simulink model "BIT8_COMP"  (R2019b)
settings: Solver=ode8  StartTime=0.0  StopTime=9999  FixedStep=1  RelTol=1e-3
values from neighbouring files (symbols this model uses):
  CODE = [ ... (first row only)    [ATE_BIT_SCRIPTS.m]
libraries: TURING_LOGIC x44, NOT x2
settings Model: EnablePacing=on  Creator=JTHURT  LastModifiedBy=JTHURT
settings DebuggingCC: SFMachineParentedDataDiag=error

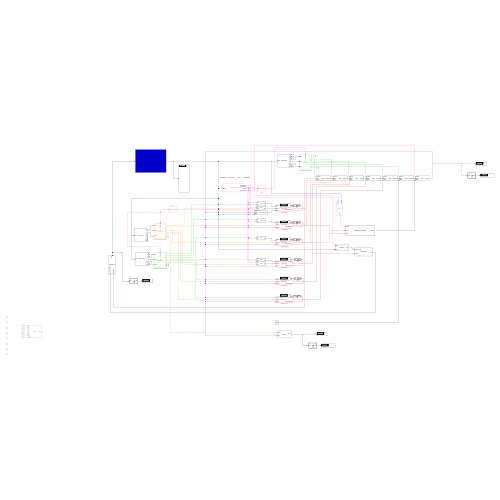
[thumbnail: Simulink's stored preview of the top-level diagram]
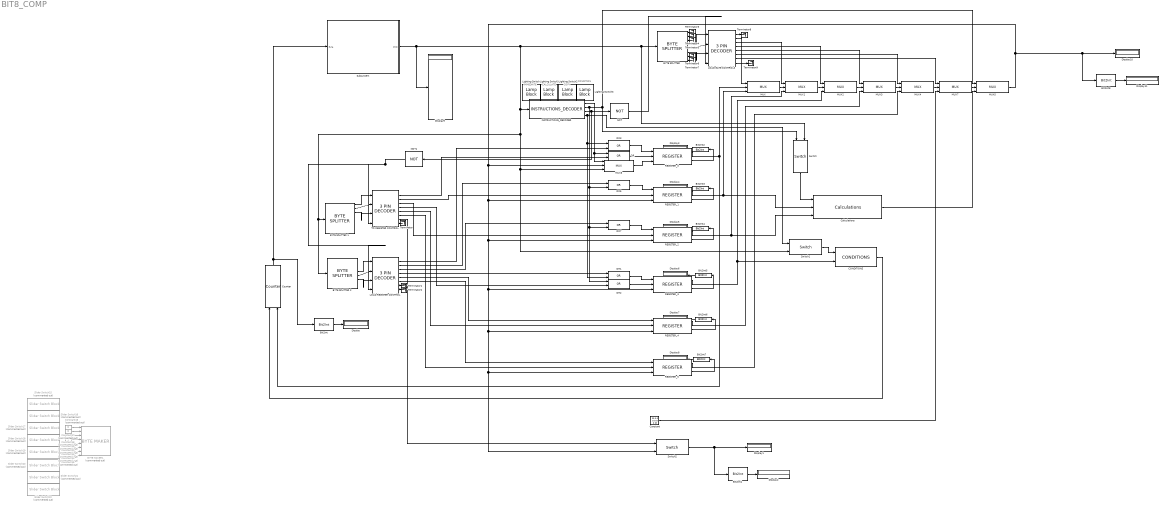
== system BIT8_COMP ==
  note: CONDITION
  note: COPY
  note: CALCULATE
  note: IMMEDIATE
  BYTE MAKER1 : TURING_LOGIC/BYTE MAKER  Commented=on  SystemSampleTime=-1  Latency=0  AutoFrameSizeCalculation=off
      settings: SourceProductName=Turing Logic
  "BYTE SPLITTER " : TURING_LOGIC/BYTE SPLITTER   SystemSampleTime=-1  Latency=0  AutoFrameSizeCalculation=off
      settings: SourceProductName=Turing Logic
  BYTE SPLITTER 1 : TURING_LOGIC/BYTE SPLITTER   SystemSampleTime=-1  Latency=0  AutoFrameSizeCalculation=off
      settings: SourceProductName=Turing Logic
  BYTE SPLITTER 2 : TURING_LOGIC/BYTE SPLITTER   SystemSampleTime=-1  Latency=0  AutoFrameSizeCalculation=off
      settings: SourceProductName=Turing Logic
  Bit2Int{,1..8} (9 alike) : TURING_LOGIC/Bit2Int  SystemSampleTime=-1  Latency=0  AutoFrameSizeCalculation=off
      settings: SourceProductName=Turing Logic
  CONDITIONS : TURING_LOGIC/CONDITIONS  SystemSampleTime=-1  Latency=0  AutoFrameSizeCalculation=off
      settings: SourceProductName=Turing Logic
  Calculations : TURING_LOGIC/Calculations  SystemSampleTime=-1  Latency=0  AutoFrameSizeCalculation=off
      settings: SourceProductName=Turing Logic
  Constant : Constant  Value=[0 0 0 0 0 0 0 0]  SampleTime=-1
  Constant{13..14,16..18,20} (6 alike) : Constant  Commented=on  Value=0  SampleTime=-1
  Constant15 : Constant  Commented=on  SampleTime=-1
  Constant19 : Constant  Commented=on  SampleTime=-1
  Counter : TURING_LOGIC/Counter  SystemSampleTime=-1  Latency=0  AutoFrameSizeCalculation=off
      settings: SourceProductName=Turing Logic
  Display{,1..11} (12 alike) : Display
  INSTRUCTIONS_DECODER : TURING_LOGIC/INSTRUCTIONS_DECODER  SystemSampleTime=-1  Latency=0  AutoFrameSizeCalculation=off
      settings: SourceProductName=Turing Logic
  LOAD GATE CONTROLS : TURING_LOGIC/3 PIN DECODER  SystemSampleTime=-1  Latency=0  AutoFrameSizeCalculation=off
      settings: SourceProductName=Turing Logic
  LOAD REGISTER CONTROL : TURING_LOGIC/3 PIN DECODER  SystemSampleTime=-1  Latency=0  AutoFrameSizeCalculation=off
      settings: SourceProductName=Turing Logic
  Lighting Switch{,1..3} (4 alike) : LampBlock  LabelPosition=Hide  Icon=LightingSwitch
  MUX{,1..7} (8 alike) : TURING_LOGIC/MUX  SystemSampleTime=-1  Latency=0  AutoFrameSizeCalculation=off
      settings: SourceProductName=Turing Logic
  NOT : NOT/NOT  SystemSampleTime=-1  Latency=0  AutoFrameSizeCalculation=off
  NOT1 : NOT/NOT  SystemSampleTime=-1  Latency=0  AutoFrameSizeCalculation=off
  OR{,1..3,5,7} (6 alike) : TURING_LOGIC/OR  SystemSampleTime=-1  Latency=0  AutoFrameSizeCalculation=off
      settings: SourceProductName=Turing Logic
  REGISTER_{0..5} (6 alike) : TURING_LOGIC/REGISTER  SystemSampleTime=-1  Latency=0  AutoFrameSizeCalculation=off
      settings: SourceProductName=Turing Logic
  Slider Switch{15..22} (8 alike) : SliderSwitchBlock  Commented=on
      settings: Values={{'Off', 'On'}, [0 1]}
  Subsystem : Subsystem
  Switch : TURING_LOGIC/Switch  SystemSampleTime=-1  Latency=0  AutoFrameSizeCalculation=off
      settings: SourceProductName=Turing Logic
  Switch1 : TURING_LOGIC/Switch  SystemSampleTime=-1  Latency=0  AutoFrameSizeCalculation=off
      settings: SourceProductName=Turing Logic
  Switch2 : TURING_LOGIC/Switch  SystemSampleTime=-1  Latency=0  AutoFrameSizeCalculation=off
      settings: SourceProductName=Turing Logic
  TO REGISTER CONTROL : TURING_LOGIC/3 PIN DECODER  SystemSampleTime=-1  Latency=0  AutoFrameSizeCalculation=off
      settings: SourceProductName=Turing Logic
  Terminator{,1..9} (10 alike) : Terminator
  wires:
  Counter/1 -> Bit2Int/1, Subsystem/1(Byte)
  Subsystem/1(CMD) -> Display9/1, Switch/2, "BYTE SPLITTER "/1, BYTE SPLITTER 2/1, BYTE SPLITTER 1/1, MUX6/3, Switch1/2, INSTRUCTIONS_DECODER/1
  "BYTE SPLITTER "/4 -> LOAD GATE CONTROLS/1
  "BYTE SPLITTER "/5 -> LOAD GATE CONTROLS/2
  "BYTE SPLITTER "/6 -> LOAD GATE CONTROLS/3
  MUX/1 -> MUX1/2
  MUX1/1 -> MUX2/2
  MUX2/1 -> MUX3/2
  MUX3/1 -> MUX4/2
  LOAD GATE CONTROLS/2 -> MUX/1
  LOAD GATE CONTROLS/3 -> MUX1/1
  LOAD GATE CONTROLS/4 -> MUX2/1
  LOAD GATE CONTROLS/5 -> MUX3/1
  LOAD GATE CONTROLS/6 -> MUX4/1
  BYTE SPLITTER 1/1 -> TO REGISTER CONTROL/1
  BYTE SPLITTER 1/2 -> TO REGISTER CONTROL/2
  BYTE SPLITTER 1/3 -> TO REGISTER CONTROL/3
  BYTE SPLITTER 2/4 -> LOAD REGISTER CONTROL/1
  BYTE SPLITTER 2/5 -> LOAD REGISTER CONTROL/2
  BYTE SPLITTER 2/6 -> LOAD REGISTER CONTROL/3
  OR/1 -> REGISTER_0/2
  INSTRUCTIONS_DECODER/1 -> MUX6/1, OR/1
  TO REGISTER CONTROL/1 -> OR/2
  MUX6/1 -> REGISTER_0/3
  OR5/1 -> REGISTER_1/1
  TO REGISTER CONTROL/2 -> REGISTER_1/2
  TO REGISTER CONTROL/3 -> REGISTER_2/2
  OR7/1 -> REGISTER_2/1
  OR2/1 -> REGISTER_3/2
  OR1/1 -> REGISTER_3/1
  INSTRUCTIONS_DECODER/2 -> OR2/1, OR7/2, OR5/2, MUX5/1, Switch/1
  TO REGISTER CONTROL/4 -> OR2/2
  TO REGISTER CONTROL/5 -> REGISTER_4/2
  TO REGISTER CONTROL/6 -> REGISTER_5/2
  LOAD REGISTER CONTROL/2 -> OR5/1
  LOAD REGISTER CONTROL/3 -> OR7/1
  LOAD REGISTER CONTROL/4 -> OR1/1
  LOAD REGISTER CONTROL/5 -> REGISTER_4/1
  LOAD REGISTER CONTROL/6 -> REGISTER_5/1
  REGISTER_0/1 -> Counter/2, MUX/2
  REGISTER_4/1 -> MUX3/3
  REGISTER_5/1 -> MUX4/3
  INSTRUCTIONS_DECODER/3 -> NOT1/1, NOT/1
  NOT/1 -> LOAD GATE CONTROLS/4
  Switch/1 -> Calculations/1
  Constant20/1 -> BYTE MAKER1/5
  Constant15/1 -> BYTE MAKER1/8
  Constant17/1 -> BYTE MAKER1/2
  Constant19/1 -> BYTE MAKER1/4
  Constant13/1 -> BYTE MAKER1/6
  Constant18/1 -> BYTE MAKER1/3
  Constant16/1 -> BYTE MAKER1/1
  Constant14/1 -> BYTE MAKER1/7
  MUX4/1 -> MUX7/2
  LOAD GATE CONTROLS/7 -> MUX7/1
  MUX7/1 -> MUX5/2
  Calculations/1 -> MUX5/3
  Switch1/1 -> CONDITIONS/1
  INSTRUCTIONS_DECODER/4 -> OR1/2, OR3/1, Switch1/1
  CONDITIONS/1 -> Counter/1
  OR3/1 -> REGISTER_0/1
  LOAD REGISTER CONTROL/1 -> OR3/2
  Constant/1 -> MUX7/3
  TO REGISTER CONTROL/7 -> Switch2/1
  Bit2Int/1 -> Display/1
  Switch2/1 -> Bit2Int1/1, Display1/1
  Bit2Int1/1 -> Display2/1
  Bit2Int2/1 -> Display3/1
  REGISTER_1/1 -> Calculations/2, MUX/3
  Bit2Int3/1 -> Display4/1
  REGISTER_2/1 -> Calculations/3, MUX1/3
  Bit2Int4/1 -> Display5/1
  Bit2Int5/1 -> Display6/1
  REGISTER_3/1 -> CONDITIONS/2, MUX2/3
  Bit2Int6/1 -> Display7/1
  Bit2Int7/1 -> Display8/1
  Bit2Int8/1 -> Display11/1
  MUX5/1 -> Bit2Int8/1, Display10/1, MUX6/2, REGISTER_2/3, REGISTER_4/3, Switch2/2, REGISTER_5/3, REGISTER_3/3, REGISTER_1/3
  REGISTER_0/2 -> Bit2Int2/1
  REGISTER_1/2 -> Bit2Int3/1
  REGISTER_2/2 -> Bit2Int4/1
  REGISTER_3/2 -> Bit2Int5/1
  REGISTER_4/2 -> Bit2Int6/1
  REGISTER_5/2 -> Bit2Int7/1
  NOT1/1 -> LOAD REGISTER CONTROL/4, TO REGISTER CONTROL/4
  TO REGISTER CONTROL/8 -> Terminator/1
  LOAD REGISTER CONTROL/7 -> Terminator1/1
  LOAD REGISTER CONTROL/8 -> Terminator2/1
  "BYTE SPLITTER "/1 -> Terminator3/1
  "BYTE SPLITTER "/2 -> Terminator4/1
  "BYTE SPLITTER "/3 -> Terminator5/1
  "BYTE SPLITTER "/7 -> Terminator6/1
  "BYTE SPLITTER "/8 -> Terminator7/1
  LOAD GATE CONTROLS/1 -> Terminator8/1
  LOAD GATE CONTROLS/8 -> Terminator9/1

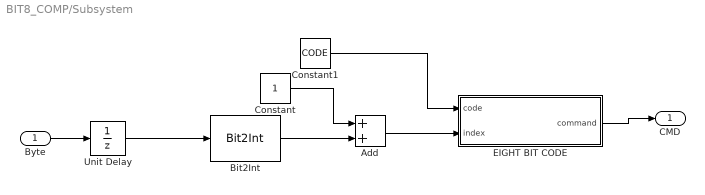
== system BIT8_COMP/Subsystem ==
  Byte : Inport
  Add : Sum
  Bit2Int : TURING_LOGIC/Bit2Int  SystemSampleTime=-1  Latency=0  AutoFrameSizeCalculation=off
      settings: SourceProductName=Turing Logic
  Constant : Constant  SampleTime=-1
  Constant1 : Constant  Value=CODE  SampleTime=-1
  EIGHT BIT CODE : MATLAB Function  TreatAsAtomicUnit=on
  Unit Delay : UnitDelay  InitialCondition=[0 0 0 0 0 0 0 0]  SampleTime=-1  HasFrameUpgradeWarning=on
  CMD : Outport
  wires:
  EIGHT BIT CODE/1(command) -> CMD/1
  Constant/1 -> Add/1
  Add/1 -> EIGHT BIT CODE/2(index)
  Constant1/1 -> EIGHT BIT CODE/1(code)
  Bit2Int/1 -> Add/2
  Byte/1 -> Unit Delay/1
  Unit Delay/1 -> Bit2Int/1

== matlab function BIT8_COMP/Subsystem/EIGHT BIT CODE ==
  data: code input; index input; command output
function command = EIGHT_BIT_CODE(code,index)

if size(code,1)> index
command = code(index,:);
else
command = code(end,:);
end 


end
